simulink model "ModellKretsVDahlberg"  (R2018a)
settings: Solver=VariableStepAuto  StartTime=0.0  StopTime=10.0  RelTol=1e-3
values from neighbouring files (symbols this model uses):
  C = 1e-4    (= 0.0001)    [SimVDahlbergsKrets.m]
  gamma = M*g/(k*C)    (= 294)    [SimVDahlbergsKrets.m]
  L = 1.5e-6    (= 1.5e-06)    [SimVDahlbergsKrets.m]
  Rx = sqrt(L/(C*k*(m+M)))*c    [SimVDahlbergsKrets.m]
settings Model: Creator=Vilmer Dahlberg  LastModifiedBy=Vilmer Dahlberg

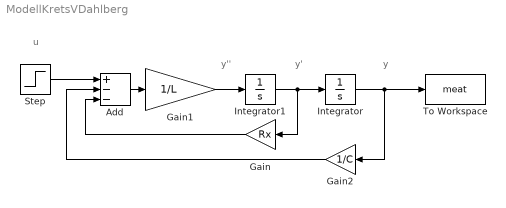
== system ModellKretsVDahlberg ==
  note: u
  note: y
  note: y'
  note: y''
  Add : Sum  Inputs=+--
  Gain : Gain  Gain=Rx
  Gain1 : Gain  Gain=1/L
  Gain2 : Gain  Gain=1/C
  Integrator : Integrator  ContinuousStateAttributes='Position'
  Integrator1 : Integrator  ContinuousStateAttributes='Velocity'
  Step : Step  Time=0  After=gamma  SampleTime=0
  To Workspace : ToWorkspace  VariableName=meat  SaveFormat=Timeseries  SampleTime=-1
  wires:
  Integrator1/1 -> Gain/1, Integrator/1
  Integrator/1 -> Gain2/1, To Workspace/1
  Gain2/1 -> Add/2
  Gain/1 -> Add/3
  Add/1 -> Gain1/1
  Gain1/1 -> Integrator1/1
  Step/1 -> Add/1
